simulink subsystem "feed_lin_double_deriv_sub"  (R2022b)
settings: Solver=VariableStepAuto  StartTime=0.0  StopTime=10.0  RelTol=1e-3
undefined symbols (not defined in the file or in its folder): double_deriv_Kd, double_deriv_Kp, wf
settings Model: Creator=Edp  LastModifiedBy=Edp

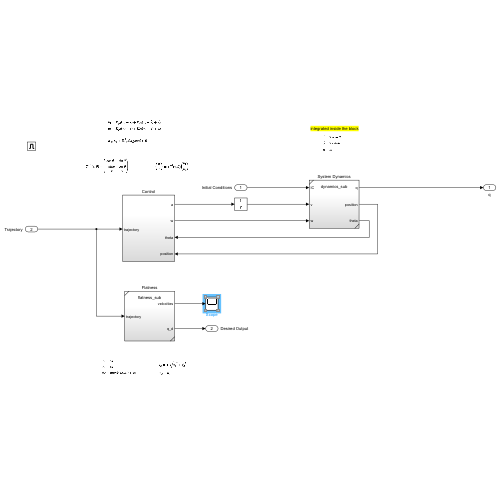
[thumbnail: Simulink's stored preview of the top-level diagram]
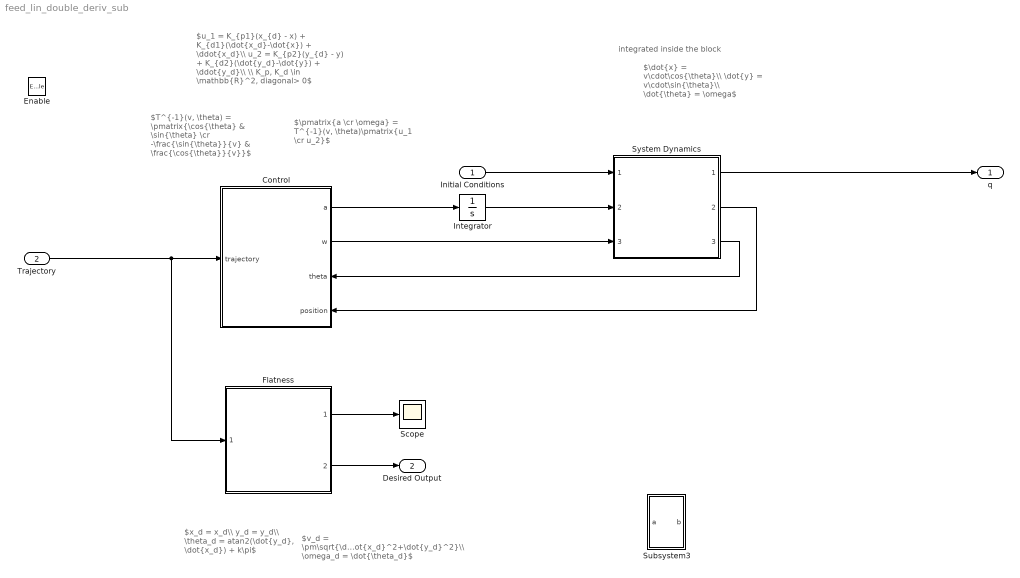
== system feed_lin_double_deriv_sub ==
  note: $u_1 = K_{p1}(x_{d} - x) + K_{d1}(\dot{x_d}-\dot{x}) + \ddot{x_d}\\ u_2 = K_{p2}(y_{d} - y) + K_{d2}(\dot{y_d}-\dot{y}) + \ddot{y_d}\\ \\ K_p, K_d \in \mathbb{R}^2, diagonal> 0$
  note: $T^{-1}(v, \theta) = \pmatrix{\cos{\theta} & \sin{\theta} \cr -\frac{\sin{\theta}}{v} & \frac{\cos{\theta}}{v}}$
  note: $\pmatrix{a \cr \omega} = T^{-1}(v, \theta)\pmatrix{u_1 \cr u_2}$
  note: $x_d = x_d\\ y_d = y_d\\ \theta_d = atan2(\dot{y_d}, \dot{x_d}) + k\pi$
  note: $v_d = \pm\sqrt{\dot{x_d}^2+\dot{y_d}^2}\\ \omega_d = \dot{\theta_d}$
  note: $\dot{x} = v\cdot\cos{\theta}\\ \dot{y} = v\cdot\sin{\theta}\\ \dot{\theta} = \omega$
  note: integrated inside the block
  Initial Conditions : Inport
  Trajectory : Inport  Port=2
  Enable : EnablePort
  Control : Subsystem
      settings: PortSchema="{\"entries\":[{\"content\":{\"sides\":[{\"content\":{\"connectorIds\":[\"In1\"]},\"type\":\"ConnectorPlacement.EquallySpacedRectSide\",\"uuid\":\"ece26907-e9a7-4b3d-a195-e49d6bc4eae1\"},{\"content\":{\"connectorIds\":[\"Out1\",\"Out2\",\"In2\",\"In3\"],\"side\":\"RIGHT\"},\"type\":\"ConnectorPlacement.EquallySpacedRectSide\",\"uuid\":\"76d01548-fb9f-437a-b1dd-300555e989a8\"},{\"content\":{\"connectorIds\":[],\"side\":\"TOP\"},\"type\":\"ConnectorPlacement.EquallySpacedRectSide\",\"uuid\":\"53f141fb-8a7f-4701-96ed-311ac642a559\"}]},\"type\":\"ConnectorPlacement.EquallySpacedConnector\",\"uuid\":\"7b949956-6c4a-4394-9731-883c67059468\"}],\"packageUris\":[\"http://schema.mathworks.com/mf0/Connector/R2020b\"],\"version\":\"1.0\"}"
  Flatness : Subsystem  ReferencedSubsystem=flatness_sub
  Integrator : Integrator
  Scope : Scope
  Subsystem3 : Subsystem
  System Dynamics : Subsystem  ReferencedSubsystem=dynamics_sub
  q : Outport
  Desired Output : Outport  Port=2
  wires:
  Flatness/1 -> Scope/1
  Control/1(a) -> Integrator/1
  System Dynamics/3 -> Control/2(theta)
  System Dynamics/2 -> Control/3(position)
  Initial Conditions/1 -> System Dynamics/1
  System Dynamics/1 -> q/1
  Flatness/2 -> Desired Output/1
  Trajectory/1 -> Control/1(trajectory), Flatness/1
  Integrator/1 -> System Dynamics/2
  Control/2(w) -> System Dynamics/3

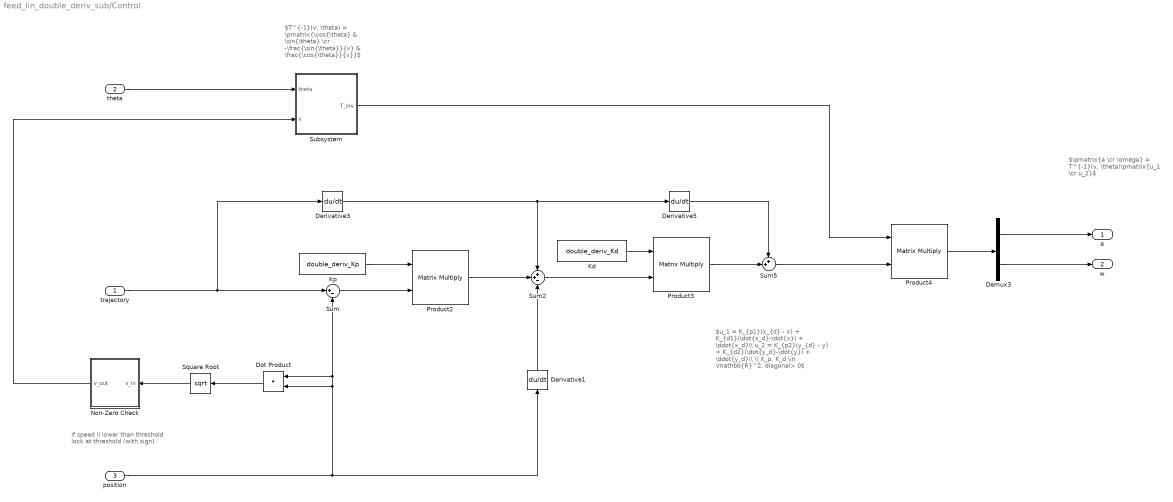
== system feed_lin_double_deriv_sub/Control ==
  note: $u_1 = K_{p1}(x_{d} - x) + K_{d1}(\dot{x_d}-\dot{x}) + \ddot{x_d}\\ u_2 = K_{p2}(y_{d} - y) + K_{d2}(\dot{y_d}-\dot{y}) + \ddot{y_d}\\ \\ K_p, K_d \in \mathbb{R}^2, diagonal> 0$
  note: $\pmatrix{a \cr \omega} = T^{-1}(v, \theta)\pmatrix{u_1 \cr u_2}$
  note: $T^{-1}(v, \theta) = \pmatrix{\cos{\theta} & \sin{\theta} \cr -\frac{\sin{\theta}}{v} & \frac{\cos{\theta}}{v}}$
  note: if speed il lower than threshold
      | lock at threshold (with sign)
  trajectory : Inport
  theta : Inport  Port=2
  position : Inport  Port=3
  Demux3 : Demux  Outputs=2
  Derivative1 : Derivative  CoefficientInTFapproximation=H
  Derivative3 : Derivative  CoefficientInTFapproximation=H
  Derivative5 : Derivative  CoefficientInTFapproximation=H
  Dot Product : DotProduct  OutDataTypeStr=Inherit: Inherit via internal rule
  Kd : Constant  Value=double_deriv_Kd
  Kp : Constant  Value=double_deriv_Kp
  Non-Zero Check : MATLAB Function  TreatAsAtomicUnit=on
  Product2 : Product  Multiplication=Matrix(*)
  Product3 : Product  Multiplication=Matrix(*)
  Product4 : Product  Multiplication=Matrix(*)
  Square Root : Sqrt
  Subsystem : Subsystem
  Sum : Sum  Inputs=|+-
  Sum2 : Sum  Inputs=++-
  Sum5 : Sum  Inputs=++|
  a : Outport
  w : Outport  Port=2
  wires:
  Derivative1/1 -> Sum2/3
  Demux3/2 -> w/1
  Demux3/1 -> a/1
  Subsystem/1(T_inv) -> Product4/1
  Product3/1 -> Sum5/2
  Sum/1 -> Product2/2
  Product2/1 -> Sum2/2
  Dot Product/1 -> Square Root/1
  Product4/1 -> Demux3/1
  Sum2/1 -> Product3/2
  Derivative5/1 -> Sum5/1
  Kd/1 -> Product3/1
  trajectory/1 -> Sum/1, Derivative3/1
  Non-Zero Check/1(v_out) -> Subsystem/2(v)
  position/1 -> Derivative1/1, Sum/2, Dot Product/1, Dot Product/2
  Derivative3/1 -> Sum2/1, Derivative5/1
  Sum5/1 -> Product4/2
  theta/1 -> Subsystem/1(theta)
  Kp/1 -> Product2/1
  Square Root/1 -> Non-Zero Check/1(v_in)

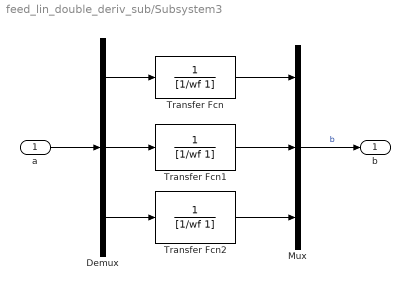
== system feed_lin_double_deriv_sub/Subsystem3 ==
  a : Inport
  Demux : Demux  Outputs=3
  Mux : Mux  Inputs=3
  Transfer Fcn : TransferFcn  Denominator=[1/wf 1]
  Transfer Fcn1 : TransferFcn  Denominator=[1/wf 1]
  Transfer Fcn2 : TransferFcn  Denominator=[1/wf 1]
  b : Outport
  wires:
  Demux/3 -> Transfer Fcn2/1
  Mux/1 -> b/1  "b"
  Demux/1 -> Transfer Fcn/1
  Transfer Fcn/1 -> Mux/1
  Transfer Fcn1/1 -> Mux/2
  Transfer Fcn2/1 -> Mux/3
  Demux/2 -> Transfer Fcn1/1
  a/1 -> Demux/1

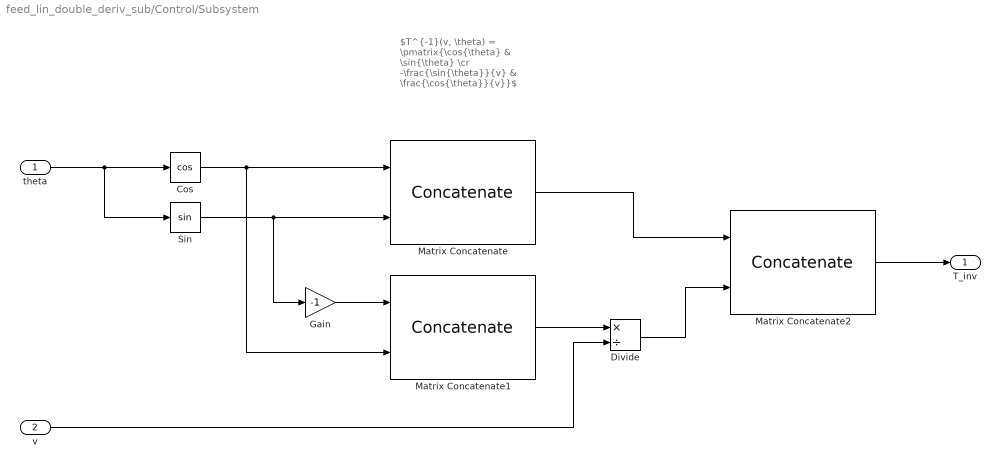
== system feed_lin_double_deriv_sub/Control/Subsystem ==
  note: $T^{-1}(v, \theta) = \pmatrix{\cos{\theta} & \sin{\theta} \cr -\frac{\sin{\theta}}{v} & \frac{\cos{\theta}}{v}}$
  theta : Inport
  v : Inport  Port=2
  Cos : Trigonometry  Operator=cos
  Divide : Product  Inputs=*/
  Gain : Gain  Gain=-1
  Matrix Concatenate : Concatenate  Mode=Multidimensional array  ConcatenateDimension=2
  Matrix Concatenate1 : Concatenate  Mode=Multidimensional array  ConcatenateDimension=2
  Matrix Concatenate2 : Concatenate  Mode=Multidimensional array
  Sin : Trigonometry
  T_inv : Outport
  wires:
  theta/1 -> Sin/1, Cos/1
  Cos/1 -> Matrix Concatenate1/2, Matrix Concatenate/1
  Sin/1 -> Gain/1, Matrix Concatenate/2
  Gain/1 -> Matrix Concatenate1/1
  Matrix Concatenate1/1 -> Divide/1
  v/1 -> Divide/2
  Matrix Concatenate/1 -> Matrix Concatenate2/1
  Divide/1 -> Matrix Concatenate2/2
  Matrix Concatenate2/1 -> T_inv/1

== matlab function feed_lin_double_deriv_sub/Control/Non-Zero Check ==
  data: v_in input; v_out output
function v_out = fcn(v_in)

if abs(v_in) < 1e-4
    if v_in >= 0 
        v_out = 1e-4;
    else 
        v_out = -1e-4;
    end
else
    v_out = v_in;
end
